simulink model "robot_speed"  (R2025b)
settings: Solver=VariableStepAuto  StartTime=0.0  StopTime=10.0  RelTol=1e-3
libraries: fuzblock x1
settings Model: Creator=l0tys  LastModifiedBy=l0tys

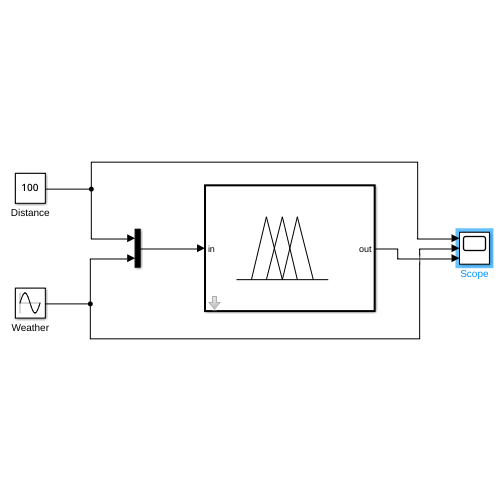
[thumbnail: Simulink's stored preview of the top-level diagram]
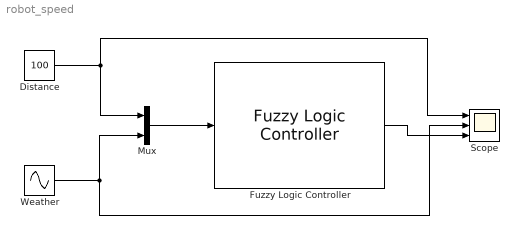
== system robot_speed ==
  Distance : Constant  Value=100
  Fuzzy Logic Controller : fuzblock/Fuzzy Logic  Controller  FIS='fuzzy_speed.fis'  OutputSampleNumber=101  DataType=double  UseLookupTable=off  NumBreakpoints=10  FuzzifiedInputs=off  RuleFiringStrengths=off  RuleOutputs=off  AggregatedOutputs=off  SimulateUsing=Interpreted execution  OutOfRangeInputValueMessage=warning  NoRuleFiredMessage=warning  EmptyOutputFuzzySetMessage=warning
  Mux : Mux  Inputs=2
  Scope : Scope  NumInputPorts=3
      settings: ActiveDisplayYMinimum=-8.9098305962793063  ActiveDisplayYMaximum=116.71458567449476
  Weather : Sin  Amplitude=50  Bias=50  SampleTime=0
  wires:
  Distance/1 -> Scope/1, Mux/1
  Weather/1 -> Scope/2, Mux/2
  Mux/1 -> Fuzzy Logic Controller/1
  Fuzzy Logic Controller/1 -> Scope/3
